simulink model "OFDM_system_QPSKmod_2024b"  (R2024b)
settings: Solver=VariableStepDiscrete  StartTime=0.0  StopTime=inf  RelTol=1e-3  EnableMultiTasking=on
PreLoadFcn:
  | EsNo=5;
  | h=[1 1]/sqrt(2);
values from neighbouring files (symbols this model uses):
  K = input('Enter the number of carriers (power of two, greater than 4):')    [run_OFDM_2011b.m]    (also in run_OFDM_2024b.m)
  seed = input('Enter the last five digits of your student ID: ')    [run_OFDM_2011b.m]    (also in run_OFDM_2024b.m; run_RAKE_Rayleigh_2021b.m = input('Enter your student ID: '); run_RAKE_Rayleigh_2024b.m = input('Enter your student ID: '))
undefined symbols (not defined in the file or in its folder): dfilt, magnitude
libraries: dspxfrm3 x3, dspobslib x3, commchan3 x2, commdigbbndpm3 x2, commrandsrc3 x1, commsink2 x1
settings Model: Creator=morelos_zaragoza  LastModifiedBy=14083
settings SolverCC: AlgebraicLoopSolver=TrustRegion
settings DataIOCC: LimitDataPoints=on  SaveFormat=Array  SignalLoggingSaveFormat=ModelDataLogs  ReturnWorkspaceOutputs=off
settings OptimizationCC: ExpressionDepthLimit=2147483647  InitFltsAndDblsToZero=on  LifeSpan=inf
settings DebuggingCC: SaveWithParameterizedLinksMsg=none  UnderspecifiedInitializationDetection=Classic  MergeDetectMultiDrivingBlocksExec=none  SignalResolutionControl=TryResolveAllWithWarning  SolverPrmCheckMsg=warning  MultiTaskDSMMsg=warning  MultiTaskCondExecSysMsg=none  FcnCallInpInsideContextMsg=warning  UnconnectedInputMsg=warning  UnconnectedOutputMsg=warning  UnconnectedLineMsg=warning  StateNameClashWarn=warning  SFUnexpectedBacktrackingDiag=warning  SFNoUnconditionalDefaultTransitionDiag=warning  SFExecutionAtInitializationDiag=none  ArithmeticOperatorsInVariantConditions=warning
settings HardwareCC: ProdBitPerPointer=32  ProdBitPerSizeT=32  ProdBitPerPtrDiffT=32  ProdLargestAtomicFloat=None  ProdIntDivRoundTo=Undefined  ProdEndianess=Unspecified  ProdWordSize=32  ProdHWDeviceType=32-bit Generic
settings ModelReferenceCC: PropagateSignalLabelsOutOfModel=off
settings SFSimCC: SimUseLocalCustomCode=off  CustomCodeUndefinedFunction=UseInterfaceOnly
settings RTWCC: RTWUseLocalCustomCode=off  GPUComputeCapability=3.5
settings CodeAppCC: StateflowObjectComments=on
settings GRTTargetCC: TargetFcnLib=ansi_tfl_tmw.mat  TargetLangStandard=C89/C90 (ANSI)  CombineOutputUpdateFcns=off  GRTInterface=on
settings ConfigComp: CovMetricSettings=dw  CovSaveCumulativeToWorkspaceVar=on  CovSaveSingleToWorkspaceVar=on  CovExternalEMLEnable=off

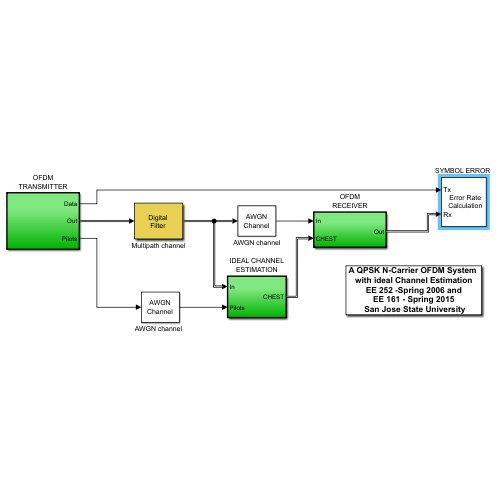
[thumbnail: Simulink's stored preview of the top-level diagram]
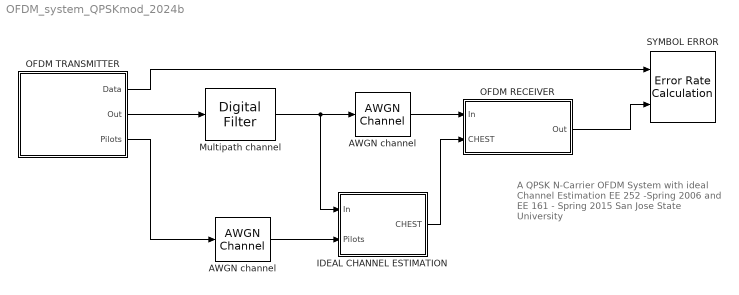
== system OFDM_system_QPSKmod_2024b ==
  note: A QPSK N-Carrier OFDM System
      | with ideal Channel Estimation
      | EE 252 -Spring 2006 and
      | EE 161 - Spring 2015
      |  San Jose State University
  AWGN channel : commchan3/AWGN Channel  LegacyMode=on  NoiseMethod="Signal to noise ratio  (SNR)"  noiseMode="Signal to noise ratio  (Es/No)"  EbNo=7  EsNo=SNR  SNR=30  BitsPerSymbol=3  SignalPower=1/K  SamplesPerSymbol=1  SymbolPeriod=1e-6/K  VarianceSource=Parameter  Variance=1  RandomStream=Global stream  Seed=seed  SimulateUsing=Code generation
  "AWGN channel  " : commchan3/AWGN Channel  LegacyMode=on  NoiseMethod="Signal to noise ratio  (SNR)"  noiseMode="Signal to noise ratio  (Es/No)"  EbNo=7  EsNo=SNR  SNR=30  BitsPerSymbol=3  SignalPower=1/K  SamplesPerSymbol=1  SymbolPeriod=1e-6/K  VarianceSource=Parameter  Variance=1  RandomStream=Global stream  Seed=6713421  SimulateUsing=Code generation
  IDEAL CHANNEL ESTIMATION : Subsystem  TreatAsAtomicUnit=on
  Multipath channel : dspobslib/Digital Filter  TypePopup=FIR (all zeros)  IIRFiltStruct=Direct form II transposed  AllPoleFiltStruct=Direct form  FIRFiltStruct=Direct form  CoeffSource=Specify via dialog  NumCoeffs=h  DenCoeffs=[1 0.1]  BiQuadCoeffs=[1 0.3 0.4 1 0.1 0.2]  LatticeCoeffs=[0.2 0.4]  denIgnore=on  FiltPerSampPopup=One filter per frame  IC=0  ICnum=0  ICden=0  roundingMode=Floor  overflowMode=off  ScaleValues=1  scaleValueFracLength=14  stageInFracLength=15  stageOutFracLength=15  FilterSource=Specify via dialog  dfiltObjectName=dfilt.dffir([1 2 1])  InputProcessing=Inherited (this choice will be removed - see release notes)
  OFDM RECEIVER : Subsystem  TreatAsAtomicUnit=on
  OFDM TRANSMITTER : Subsystem  TreatAsAtomicUnit=on
  "SYMBOL ERROR " : commsink2/Error Rate Calculation  N=0  st_delay=K  cp_mode=Entire frame  subframe=[]  PMode=Workspace  WsName=ErrorVec  RsMode2=off  stop=on  numErr=500  maxBits=1000000
  wires:
  Multipath channel/1 -> AWGN channel/1, IDEAL CHANNEL ESTIMATION/1(In)
  OFDM RECEIVER/1(Out) -> "SYMBOL ERROR "/2
  OFDM TRANSMITTER/2(Out) -> Multipath channel/1
  OFDM TRANSMITTER/1(Data) -> "SYMBOL ERROR "/1
  OFDM TRANSMITTER/3(Pilots) -> "AWGN channel  "/1
  AWGN channel/1 -> OFDM RECEIVER/1(In)
  IDEAL CHANNEL ESTIMATION/1(CHEST) -> OFDM RECEIVER/2(CHEST)
  "AWGN channel  "/1 -> IDEAL CHANNEL ESTIMATION/2(Pilots)

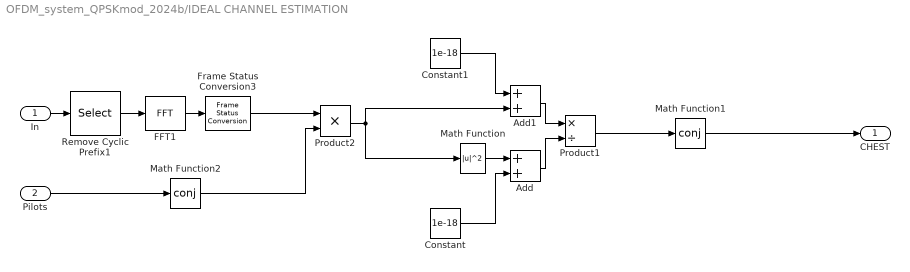
== system OFDM_system_QPSKmod_2024b/IDEAL CHANNEL ESTIMATION ==
  In : Inport
  Pilots : Inport  Port=2
  Add : Sum
  Add1 : Sum
  Constant : Constant  Value=1e-18  VectorParams1D=off
  Constant1 : Constant  Value=1e-18  VectorParams1D=off
  FFT1 : dspxfrm3/FFT  FFTImplementation=Auto  CompMethod=Table lookup  TableOpt=HYBRID  TableOptActive=Speed  BitRevOrder=off  Normalize=off  InheritFFTLength=on  FFTLength=64  WrapInput=on  roundingMode=Floor  overflowMode=off  firstCoeffDataTypeStr=Inherit: Same word length as input  firstCoeffLastDataTypeStr=Inherit: Same word length as input  outputMin=[]  outputMax=[]
  Frame Status Conversion3 : dspobslib/Frame Status Conversion  growRefPort=off  outframe=Frame-based
  Math Function : Math  Operator=magnitude^2  SignedPower=on
  Math Function1 : Math  Operator=conj  SignedPower=on
  Math Function2 : Math  Operator=conj  SignedPower=on
  Product1 : Product  Inputs=*/  RndMeth=Zero
  Product2 : Product  RndMeth=Zero
  Remove Cyclic Prefix1 : Selector  InputPortWidth=5*K/4  IndexOptions=Index vector (dialog)  Indices=[K/4+1:5*K/4]  OutputSizes=1
  CHEST : Outport
  wires:
  FFT1/1 -> Frame Status Conversion3/1
  Remove Cyclic Prefix1/1 -> FFT1/1
  Product1/1 -> Math Function1/1
  Product2/1 -> Math Function/1, Add1/2
  Frame Status Conversion3/1 -> Product2/1
  Math Function2/1 -> Product2/2
  Math Function/1 -> Add/1
  Constant/1 -> Add/2
  Add/1 -> Product1/2
  Constant1/1 -> Add1/1
  Add1/1 -> Product1/1
  Pilots/1 -> Math Function2/1
  In/1 -> Remove Cyclic Prefix1/1
  Math Function1/1 -> CHEST/1

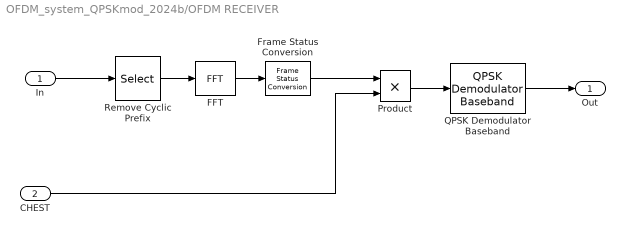
== system OFDM_system_QPSKmod_2024b/OFDM RECEIVER ==
  In : Inport
  CHEST : Inport  Port=2
  FFT : dspxfrm3/FFT  FFTImplementation=Auto  CompMethod=Table lookup  TableOpt=HYBRID  TableOptActive=Speed  BitRevOrder=off  Normalize=off  InheritFFTLength=on  FFTLength=64  WrapInput=on  roundingMode=Floor  overflowMode=off  firstCoeffDataTypeStr=Inherit: Same word length as input  firstCoeffLastDataTypeStr=Inherit: Same word length as input  outputMin=[]  outputMax=[]
  Frame Status Conversion : dspobslib/Frame Status Conversion  growRefPort=off  outframe=Frame-based
  Product : Product  RndMeth=Zero
  QPSK Demodulator Baseband : commdigbbndpm3/QPSK Demodulator Baseband  OutType=Integer  DecType=Hard decision  VarSource=Dialog  Variance=1  Dec=Gray  Ph=pi/4  outDtype1=Inherit via internal rule  outDtype2=Inherit via internal rule  derotateFactorWordLen=16  derotateFactorDataTypeStr=Inherit: Same word length as input  derotateFactorLastDataTypeStr=Inherit: Same word length as input
  Remove Cyclic Prefix : Selector  InputPortWidth=5*K/4  IndexOptions=Index vector (dialog)  Indices=[K/4+1:5*K/4]  OutputSizes=1
  Out : Outport
  wires:
  FFT/1 -> Frame Status Conversion/1
  Remove Cyclic Prefix/1 -> FFT/1
  Product/1 -> QPSK Demodulator Baseband/1
  In/1 -> Remove Cyclic Prefix/1
  Frame Status Conversion/1 -> Product/1
  CHEST/1 -> Product/2
  QPSK Demodulator Baseband/1 -> Out/1

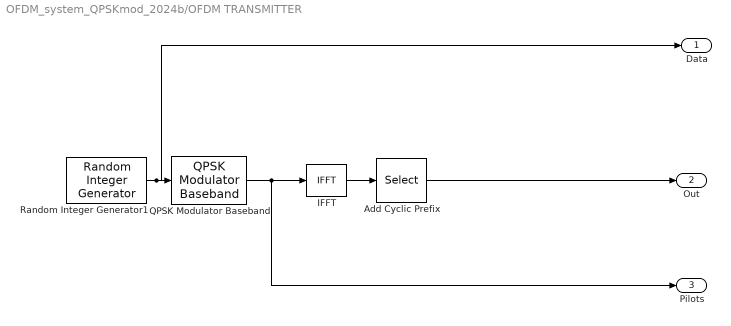
== system OFDM_system_QPSKmod_2024b/OFDM TRANSMITTER ==
  Add Cyclic Prefix : Selector  InputPortWidth=K  IndexOptions=Index vector (dialog)  Indices=[3*K/4+1:K 1:K]  OutputSizes=1
  IFFT : dspxfrm3/IFFT  FFTImplementation=Auto  CompMethod=Table lookup  TableOpt=HYBRID  TableOptActive=Speed  BitRevOrder=off  cs_in=off  Normalize=on  InheritFFTLength=on  FFTLength=64  WrapInput=on  mode=Complex  outSamplingMode=Frame based  roundingMode=Floor  overflowMode=off  firstCoeffDataTypeStr=Inherit: Same word length as input  firstCoeffLastDataTypeStr=Inherit: Same word length as input  outputMin=[]  outputMax=[]
  QPSK Modulator Baseband : commdigbbndpm3/QPSK Modulator Baseband  InType=Integer  Enc=Gray  Ph=pi/4  outDtype=double  outWordLen=16  outUDDataType=sfix(16)  outFracLenMode=Best precision  outFracLen=15  outDataTypeStr=double  outLastDataTypeStr=double
  Random Integer Generator1 : commrandsrc3/Random Integer Generator  SetSize=4  SeedSource=Parameter  Seed=seed  SampleTime=1e-6/K  SamplesPerFrame=K  OutputDataType=double  SimulateUsing=Interpreted execution
  Data : Outport
  Out : Outport  Port=2
  Pilots : Outport  Port=3
  wires:
  Random Integer Generator1/1 -> Data/1, QPSK Modulator Baseband/1
  QPSK Modulator Baseband/1 -> IFFT/1, Pilots/1
  Add Cyclic Prefix/1 -> Out/1
  IFFT/1 -> Add Cyclic Prefix/1
